simulink model "CheckMate_clipboard"  (R2013a)
settings: Solver=ode15s  StartTime=0.0  StopTime=0.5  FixedStep=1e-3  RelTol=1e-5  AbsTol=1e-8
PreLoadFcn:
  | setup5d,etc_def
undefined symbols (not defined in the file): alpha_des, red_fil, surfA, surfB
libraries: cmlib x10
settings Model: ExtModeTrigMode=oneshot  ExtModeArmWhenConnect=off  Creator=zhan  LastModifiedBy=zhan
settings DataIOCC: LimitDataPoints=off  SignalLoggingSaveFormat=ModelDataLogs  SignalLoggingName=sigsOut
settings OptimizationCC: BlockReduction=off
settings DebuggingCC: SaveWithParameterizedLinksMsg=none  SignalResolutionControl=TryResolveAllWithWarning  SolverPrmCheckMsg=none  MultiTaskDSMMsg=warning  MultiTaskCondExecSysMsg=none  StrictBusMsg=None
settings HardwareCC: TargetUnknown=on
settings SFSimCC: SimParseCustomCode=off
settings RTWCC: IncludeERTFirstTime=on
settings GRTTargetCC: CombineOutputUpdateFcns=off  GRTInterface=on

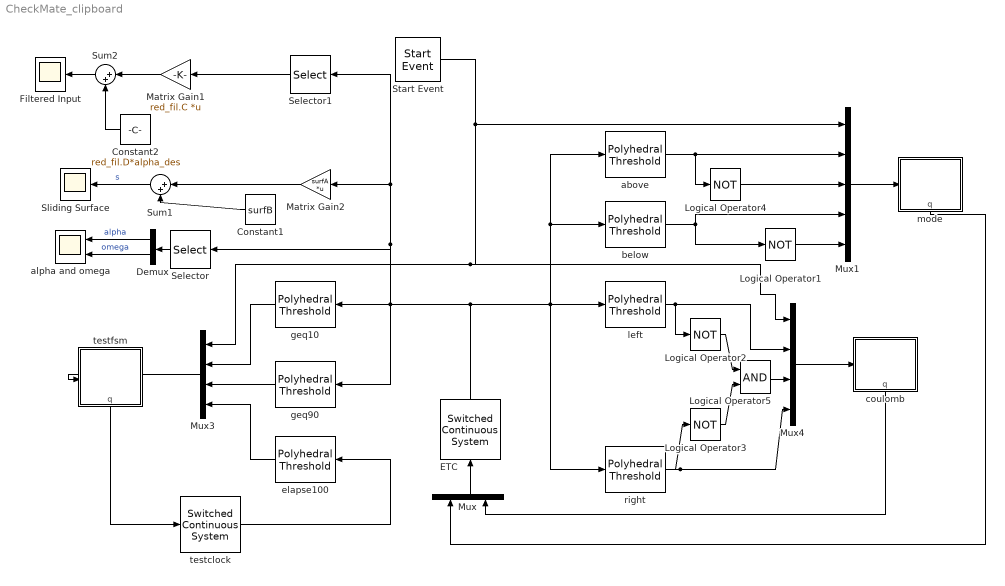
== system CheckMate_clipboard ==
  Constant1 : Constant  Value=surfB
  Constant2 : Constant  Value=red_fil.D*alpha_des
  Demux : Demux  Outputs=2
  ETC : cmlib/Switched Continuous System  nx=4  use_sd=off  nup=[]  nz=[]  use_reset=off  nu=2  x0=[0;0;0;0]  swfunc=slidingmode  ICS=etc_ICS  AR=etc_AR  use_param=on  p0=[1.2;1.2]  PaCs=etc_PaCs
  Filtered Input : Scope
      settings: TimeRange=0.5  YMin=-0.5  YMax=2
  Logical Operator{1..4} (4 alike) : Logic  Operator=NOT
  Logical Operator5 : Logic
  Matrix Gain1 : Gain  Gain=red_fil.C  Multiplication=Matrix(K*u)  SaturateOnIntegerOverflow=on  OutDataTypeStr=Inherit: Same as input  ParamDataTypeStr=Inherit: Same as input
  Matrix Gain2 : Gain  Gain=surfA  Multiplication=Matrix(K*u)  SaturateOnIntegerOverflow=on  OutDataTypeStr=Inherit: Same as input  ParamDataTypeStr=Inherit: Same as input
  Mux : Mux  Inputs=2
  Mux1 : Mux  Inputs=5
  Mux3 : Mux
  Mux4 : Mux
  Selector : Selector  InputPortWidth=4  IndexOptions=Index vector (dialog)  Indices=[3 4]  OutputSizes=1
  Selector1 : Selector  InputPortWidth=4  IndexOptions=Index vector (dialog)  Indices=[1 2]  OutputSizes=1
  Sliding Surface : Scope
      settings: TimeRange=0.5  YMax=35  SaveName=ScopeData4
  Start Event : cmlib/Start Event  steptime=0.01  initval=0  finival=1  sampletime=0  interpret=on  enable=on
  Sum1 : Sum  Inputs=|++  SaturateOnIntegerOverflow=on  InputSameDT=on  OutDataTypeStr=Inherit: Same as first input
  Sum2 : Sum  Inputs=|++  SaturateOnIntegerOverflow=on  InputSameDT=on  OutDataTypeStr=Inherit: Same as first input
  above : cmlib/Polyhedral Threshold  polyhedron=above_surf
  alpha and omega : Scope  NumInputPorts=2
      settings: TimeRange=0.5  YMin=0~-10  YMax=2~30  SaveName=AandO  DataFormat=Structure
  below : cmlib/Polyhedral Threshold  polyhedron=below_surf
  coulomb : Stateflow chart  TreatAsAtomicUnit=on
  elapse100 : cmlib/Polyhedral Threshold  polyhedron=clock_geq100
  geq10 : cmlib/Polyhedral Threshold  polyhedron=alpha_geq10
  geq90 : cmlib/Polyhedral Threshold  polyhedron=alpha_geq90
  left : cmlib/Polyhedral Threshold  polyhedron=turn_left
  mode : Stateflow chart  TreatAsAtomicUnit=on
  right : cmlib/Polyhedral Threshold  polyhedron=turn_right
  testclock : cmlib/Switched Continuous System  nx=1  use_sd=off  nup=[]  nz=[]  use_reset=off  nu=1  x0=0  swfunc=testclock  ICS=clock_ICS  AR=clock_AR  use_param=off  p0=[]  PaCs=[]
  testfsm : Stateflow chart  TreatAsAtomicUnit=on
  wires:
  ETC/1 -> left/1, below/1, above/1, right/1, geq90/1, Matrix Gain2/1, Selector1/1, Selector/1, geq10/1
  Mux/1 -> ETC/1
  mode/1(q) -> Mux/1
  Matrix Gain2/1 -> Sum1/1
  Constant1/1 -> Sum1/2
  Sum1/1 -> Sliding Surface/1  "s"
  Mux4/1 -> coulomb/Trigger
  left/1 -> Mux4/2, Logical Operator2/1
  right/1 -> Mux4/4, Logical Operator3/1
  Mux1/1 -> mode/Trigger
  Logical Operator1/1 -> Mux1/5
  Logical Operator4/1 -> Mux1/3
  below/1 -> Logical Operator1/1, Mux1/4
  above/1 -> Logical Operator4/1, Mux1/2
  coulomb/1(q) -> Mux/2
  Start Event/1 -> Mux1/1, Mux4/1, Mux3/1
  Selector/1 -> Demux/1
  Demux/1 -> alpha and omega/1  "alpha"
  Demux/2 -> alpha and omega/2  "omega"
  Selector1/1 -> Matrix Gain1/1
  Sum2/1 -> Filtered Input/1
  Matrix Gain1/1 -> Sum2/1
  Constant2/1 -> Sum2/2
  testclock/1 -> elapse100/1
  Mux3/1 -> testfsm/Trigger
  testfsm/1(q) -> testclock/1
  geq10/1 -> Mux3/2
  geq90/1 -> Mux3/3
  elapse100/1 -> Mux3/4
  Logical Operator5/1 -> Mux4/3
  Logical Operator2/1 -> Logical Operator5/1
  Logical Operator3/1 -> Logical Operator5/2

== stateflow chart CheckMate_clipboard/mode ==
  state on
    entry: q=1;
  state under
    entry: q=2;
  state beyond
    entry: q=3;
  (default) -> beyond : start
  on -> beyond [order 1] : above
  on -> under [order 2] : below
  under -> on : negbelow
  beyond -> on : negabove
  data: q output int16
  events: start input RISING_EDGE_EVENT; above input RISING_EDGE_EVENT; negabove input RISING_EDGE_EVENT; below input RISING_EDGE_EVENT; negbelow input RISING_EDGE_EVENT

== stateflow chart CheckMate_clipboard/testfsm ==
  state avoid
    entry: q=3;
  state above0
    entry: q=1;
  state above10
    entry:q=2;
  state reach
    entry: q=4;
  (default) -> above0 : start
  above10 -> avoid [order 1] : elapse100
  above0 -> above10 : geq10
  above10 -> reach [order 2] : geq90
  data: q output int16
  events: start input RISING_EDGE_EVENT; geq10 input RISING_EDGE_EVENT; geq90 input RISING_EDGE_EVENT; elapse100 input RISING_EDGE_EVENT

== stateflow chart CheckMate_clipboard/coulomb ==
  state left
    entry: q=2;
  state neither
    entry: q=1;
  state right
    entry: q=3;
  (default) -> neither : start
  right -> neither : negturn
  neither -> left [order 2] : turnleft
  left -> neither : negturn
  neither -> right [order 1] : turnright
  data: q output int16
  events: start input RISING_EDGE_EVENT; turnleft input RISING_EDGE_EVENT; negturn input RISING_EDGE_EVENT; turnright input RISING_EDGE_EVENT
